simulink model "Hybrid_PV_Wind_Subsystem"  (R2018a)
settings: Solver=ode5  StartTime=0.0  StopTime=10  RelTol=1e-3
PreLoadFcn:
  | Ts_Power=1e-6;
  | Ts_Control=100e-6;
undefined symbols (not defined in the file): D1, Delta, DiscIntNeverNeededParam, sigbuilder_block
libraries: powerlib x32, powerlib_meascontrol x11, re_lib x2, simulink x2
(part 1 of 2)
Description:
  | Copyright 2008-2018 The MathWorks, Inc.
settings Model: SimulationMode=accelerator  Creator=MathWorks  LastModifiedBy=ASUS
settings DataIOCC: LimitDataPoints=on  SaveFormat=Array  SignalLoggingSaveFormat=ModelDataLogs  SignalLogging=off  DSMLogging=off
settings OptimizationCC: ExpressionDepthLimit=2147483647  EfficientMapNaN2IntZero=off  LifeSpan=inf
settings DebuggingCC: UnderspecifiedInitializationDetection=Classic  MergeDetectMultiDrivingBlocksExec=none  SolverPrmCheckMsg=warning  FcnCallInpInsideContextMsg=warning  StateNameClashWarn=warning  LibraryContextMissingDiagnostic=warning  SFUnexpectedBacktrackingDiag=warning  SFNoUnconditionalDefaultTransitionDiag=warning  SFExecutionAtInitializationDiag=none
settings HardwareCC: ProdBitPerPointer=32  ProdBitPerSizeT=32  ProdBitPerPtrDiffT=32  ProdLargestAtomicFloat=None  ProdIntDivRoundTo=Undefined  ProdEndianess=Unspecified  ProdWordSize=32  ProdHWDeviceType=32-bit Generic  TargetBitPerPointer=64  TargetBitPerSizeT=64  TargetBitPerPtrDiffT=64  TargetLongLongMode=on  TargetIntDivRoundTo=Zero  TargetEndianess=LittleEndian  TargetWordSize=64  TargetHWDeviceType=MATLAB Host  ProdEqTarget=off
settings ModelReferenceCC: PropagateSignalLabelsOutOfModel=off
settings RTWCC: RTWUseLocalCustomCode=on
settings CodeAppCC: MaxIdLength=128
settings GRTTargetCC: TargetLangStandard=C89/C90 (ANSI)  CombineOutputUpdateFcns=off  GRTInterface=on
settings ConfigComp: CovMetricSettings=dw  CovHtmlReporting=on  CovSaveCumulativeToWorkspaceVar=on  CovSaveSingleToWorkspaceVar=on  CovExternalEMLEnable=off  CovSFcnEnable=off
settings SimscapeCC: SimscapeNormalizeSystem=off

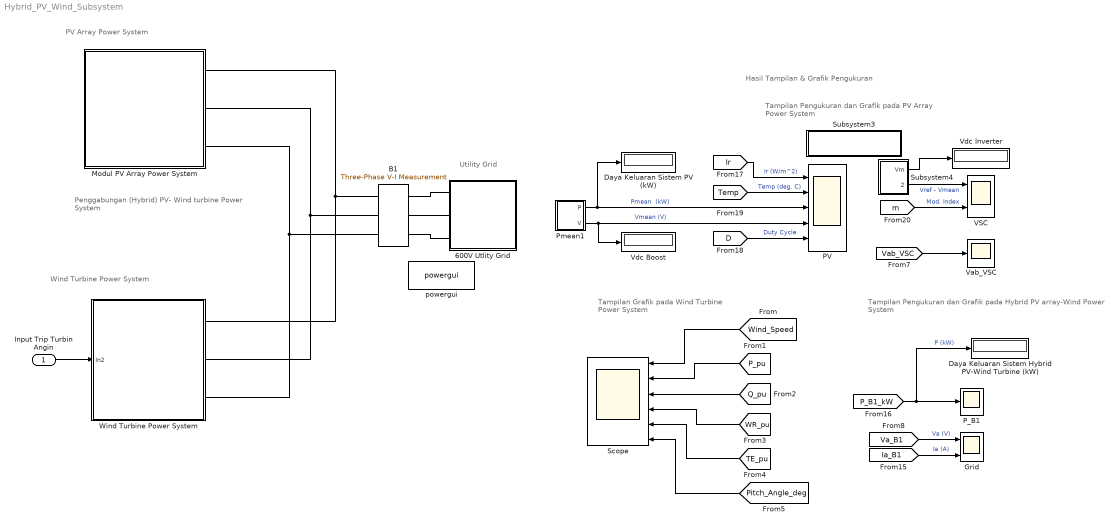
== system Hybrid_PV_Wind_Subsystem ==
  note: Hasil Tampilan & Grafik Pengukuran
  note: Penggabungan
      | (Hybrid) PV- Wind turbine
      | Power System
  note: Tampilan Grafik pada
      | Wind Turbine Power System
  note: PV Array Power System
  note: Wind Turbine Power System
  note: Tampilan Pengukuran dan
      | Grafik pada PV Array Power System
  note: Tampilan Pengukuran dan
      | Grafik pada Hybrid PV array-Wind Power System
  note: Utility Grid
  Input Trip Turbin Angin : Inport
  " Modul PV Array Power System" : Subsystem
  " Wind Turbine Power System" : Subsystem
  600V Utlity Grid : Subsystem
      mask Display: image(imread('grid.jpg'))
  B1 : powerlib/Measurements/Three-Phase V-I Measurement  VoltageMeasurement=phase-to-ground  SetLabelV=on  LabelV=Vabc_B1  Vpu=off  VpuLL=off  CurrentMeasurement=yes  SetLabelI=on  LabelI=Iabc_B1  Ipu=off  Pbase=100e6  Vbase=500e3  OutputType=Magnitude  PhasorSimulation=on  PSBequivalent=0
      settings: SourceProductName=Simscape Electrical
  Daya Keluaran Sistem Hybrid PV-Wind Turbine (kW) : Display
      settings: Format=bank  Decimation=2000
  "Daya Keluaran Sistem PV (kW) " : Display
      settings: Format=bank  Decimation=2000
  Grid : Scope  NumInputPorts=2
  PV : Scope  NumInputPorts=5
  P_B1 : Scope
  Pmean1 : Subsystem
  Scope : Scope  NumInputPorts=6
  Subsystem3 : Subsystem
      mask Display: disp('Open this block\nto display additional \nscopes & measurements')
  Subsystem4 : Subsystem
  VSC : Scope  NumInputPorts=2
  Vab_VSC : Scope
  Vdc Boost : Display
      settings: Format=bank  Decimation=2000
  Vdc Inverter : Display
      settings: Format=bank  Decimation=2000
  powergui : powerlib/powergui  Priority=1  SimulationMode=Discrete  SampleTime=Ts_Power  frequency=60  Iterations=50  frequencyindice=0  Pbase=100e6  ErrMax=1e-4  UnitsV=kV  UnitsW=MW  buscounter=0  FunctionMessages=off  echomessages=off  EnableUseOfTLC=off  CurrentSourceSwitches=off  DisableSnubberDevices=off  DisableRonSwitches=off  DisableVfSwitches=off  DisplayEquations=off  SolverType=Tustin/Backward Euler (TBE)  Interpol=off  ExternalGateDelay=off  methode=off  Ts=0  x0status=blocks  SPID=off  SwTol=0  HookPort=off  RestoreLinks=warning  ResistiveCurrentMeasurement=off  Frange=[0:2:500]  Ylog=off  Xlog=on  ShowGrid=off  save=off  variable=ZData  structure=0  ZoomFFT=on  StartTime=0.0  cycles=1  DisplayStyle=1  fundamental=60  FreqAxis=off  MaxFrequency=1000  frequencyindicesteady=1  RmsSteady=1  display=off
  wires:
  Subsystem4/2(VrVm) -> VSC/1  "Vref - Vmean"
  Pmean1/1(P) -> "Daya Keluaran Sistem PV (kW) "/1, PV/3  "Pmean  (kW)"
  [Ir] -> PV/1  "Ir (W/m^2)"
  [Ia_B1] -> Grid/2  "Ia (A)"
  [Temp] -> PV/2  "Temp (deg. C)"
  [Va_B1] -> Grid/1  "Va (V)"
  Pmean1/2(V) -> Vdc Boost/1, PV/4  "Vmean (V)"
  [D] -> PV/5  "Duty Cycle"
  [P_B1_kW] -> P_B1/1, Daya Keluaran Sistem Hybrid PV-Wind Turbine (kW)/1  "P (kW)"
  [Vab_VSC] -> Vab_VSC/1
  [m] -> VSC/2  "Mod. Index"
  Subsystem4/1(Vm) -> Vdc Inverter/1
  Input Trip Turbin Angin/1 -> " Wind Turbine Power System"/1(In2)
  [Wind_Speed] -> Scope/1
  [P_pu] -> Scope/2
  [Q_pu] -> Scope/3
  [WR_pu] -> Scope/4
  [TE_pu] -> Scope/5
  [Pitch_Angle_deg] -> Scope/6
  connections:
  B1/RConn3 -- 600V Utlity Grid/LConn3
  B1/RConn2 -- 600V Utlity Grid/LConn2
  B1/RConn1 -- 600V Utlity Grid/LConn1
  " Modul PV Array Power System"/RConn1 -- " Wind Turbine Power System"/RConn1 -- B1/LConn1
  " Modul PV Array Power System"/RConn2 -- " Wind Turbine Power System"/RConn2 -- B1/LConn2
  " Modul PV Array Power System"/RConn3 -- " Wind Turbine Power System"/RConn3 -- B1/LConn3

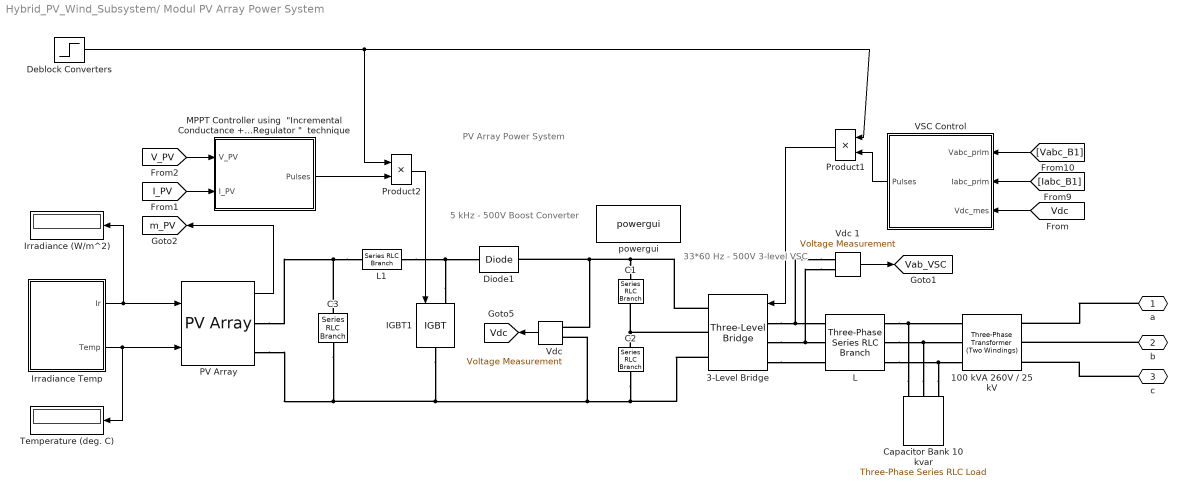
== system Hybrid_PV_Wind_Subsystem/ Modul PV Array Power System ==
  note: 5 kHz - 500V
      | Boost Converter
  note: 33*60 Hz - 500V
      | 3-level VSC
  note: PV Array Power System
  100 kVA 260V / 25 kV : powerlib/Elements/Three-Phase Transformer (Two Windings)  Winding1Connection=Yg  Winding2Connection=Delta (D1)  CoreType=Three single-phase transformers  SetSaturation=off  Hysteresis=off  DataFile='hysteresis'  SetInitialFlux=off  Measurements=None  UNITS=pu  NominalPower=[100e3 , 60 ]  Winding1=[ 25e3 , 0.001 , 0.03 ]  Winding2=[ 260 , 0.001 , 0.03 ]  Rm=500  Lm=500  L0=0.5  Saturation=[ 0,0 ; 0.0024,1.2 ; 1.0,1.52 ]  InitialFluxes=[ 0.8 , -0.8 , 0.7 ]  MoreParameters=off  BreakLoop=off  DataType=off  TransfoNumber=0
      settings: SourceProductName=Simscape Electrical
  3-Level Bridge : powerlib/Power Electronics/Three-Level Bridge  Arms=3  SnubberResistance=1e6  SbubberCapacitance=inf  Device=IGBT / Diodes  Ron=0.2e-3  ForwardVoltages="[  0  0 ]"  Measurements=None
      settings: SourceProductName=Simscape Electrical  SourceProductBaseCode=PS
  C1 : powerlib/Elements/Series RLC Branch  LConnTagsString=__new0  RConnTagsString=__new0  BranchType=C  Resistance=1.0  Inductance=1.0  SetiL0=off  InitialCurrent=0  Capacitance=12000e-06  Setx0=off  InitialVoltage=0  Measurements=None
      settings: SourceProductName=Simscape Electrical
  C2 : powerlib/Elements/Series RLC Branch  LConnTagsString=__new0  RConnTagsString=__new0  BranchType=C  Resistance=1.0  Inductance=1.0  SetiL0=off  InitialCurrent=0  Capacitance=12000e-06  Setx0=off  InitialVoltage=0  Measurements=None
      settings: SourceProductName=Simscape Electrical
  C3 : powerlib/Elements/Series RLC Branch  LConnTagsString=__new0  RConnTagsString=__new0  BranchType=C  Resistance=1.0  Inductance=1.0  SetiL0=off  InitialCurrent=0  Capacitance=100e-6  Setx0=off  InitialVoltage=0  Measurements=Branch voltage
      settings: SourceProductName=Simscape Electrical
  Capacitor Bank 10 kvar : powerlib/Elements/Three-Phase Series RLC Load  LConnTagsString=A|B|C  Configuration=Y (grounded)  NominalVoltage=240  Vabc=[1e3 1e3 1e3]  Vabcp=[1e3 1e3 1e3]  NominalFrequency=60  UnbalancedPower=off  ActivePower=10e3/100  InductivePower=0  CapacitivePower=10e3  Pabc=[10e3 9e3 11e3]  QLabc=[100 90 110]  QCabc=[100 90 110]  Pabcp=[10e3 9e3 11e3]  QLabcp=[100 90 110]  QCabcp=[100 90 110]  Measurements=None  LoadType=constant Z
      settings: SourceProductName=Simscape Electrical
  Deblock Converters : Step  Time=0.05  SampleTime=0
  Diode1 : powerlib/Power Electronics/Diode  Ron=1e-4  Lon=0  Vf=0  IC=0  UseSnubber=off  Rs=inf  Cs=inf  Measurements=off
      settings: SourceProductName=Simscape Electrical
  IGBT1 : powerlib/Power Electronics/IGBT  Ron=0.001  Lon=0  Vf=0  Tf=0  Tt=0  IC=0  Rs=1e5  Cs=inf  Measurements=off
      settings: SourceProductName=Simscape Electrical
  Irradiance (W/m^2) : Display
      settings: Format=bank  Decimation=1000
  Irradiance Temp : Subsystem  Tag=STV Subsys  LoadFcn=sigbuilder_block('load');  StartFcn=sigbuilder_block('start');  StopFcn=sigbuilder_block('stop');  ClipboardFcn=sigbuilder_block('clipboard');  mask(Sigbuilder block){tuvar=[0:10]}
      mask help: Sigbuilder GUI
      mask init:
      | if ~strcmp(get_param(bdroot(gcbh),'SimulationStatus'),'stopped') tuvar = sigbuilder_block('maskInit'); end
      settings: CopyFcn=sigbuilder_block('copy');  DeleteFcn=sigbuilder_block('delete');  ModelCloseFcn=sigbuilder_block('modelClose');  PreSaveFcn=sigbuilder_block('preSave');  PauseFcn=sigbuilder_block('pause')  ContinueFcn=sigbuilder_block('continue')  NameChangeFcn=sigbuilder_block('namechange');  OpenFcn=sigbuilder_block('open',[216.75 77.25 531 395.25 ]);  CloseFcn=sigbuilder_block('close');
      mask Display: plot(0, 0, 100, 100,[2, 2, 32, 32, 2], [68, 8, 8, 68, 68],[32, 2], [38, 38], [32, 19, 2],[53, 60, 44], [32, 17, 17, 2],[16, 16, 31, 31]);txt = getActiveGroup(gcbh);text(2, 100, txt,'verticalAlignment', 'top');
  L : powerlib/Elements/Three-Phase Series RLC Branch  LConnTagsString=A|B|C  RConnTagsString=A|B|C  BranchType=RL  Resistance=500e-6*377/50/2  Inductance=500e-6/2  Capacitance=inf  Measurements=None
      settings: SourceProductName=Simscape Electrical
  L1 : powerlib/Elements/Series RLC Branch  LConnTagsString=__new0  RConnTagsString=__new0  BranchType=RL  Resistance=0.005  Inductance=5e-3  SetiL0=off  InitialCurrent=0  Capacitance=1e-6  Setx0=off  InitialVoltage=0  Measurements=None
      settings: SourceProductName=Simscape Electrical
  "MPPT Controller using  \"Incremental Conductance + Integral Regulator \"  technique " : Subsystem  mask(Boost Control - MPPT){fc=5000, T_MPPT=200e-6, Dinit=0.5}
      mask prompts: fc "PWM switching frequency (Hz)"; T_MPPT "Time window used by MPPT control (s)"; Dinit "Initial value of duty cycle"
  PV Array : re_lib/Solar/PV Array  Npar=9  Nser=5  PlotType=array @ 1000 W/m2 & specified temperatures  S_vec="[ 1000  250 ]"  Temp_C_vec="[0 25 50  ]"  ModuleName=SunPower SPR-305E-WHT-D  PlotWhenSelected=off  Pm=305.226  Ncell=96  Voc=64.2  Isc=5.96  Vm=54.7  Im=5.58  beta_Voc_pc=-0.27269  alpha_Isc_pc=0.061745  beta_Voc=-0.17507  alpha_Isc=0.00368  IL=6.0092  I0=6.3014e-12  nI=0.94504  Rsh=269.5934  Rs=0.37152  BAL=on  Tc=Tc  Tfilter=5e-5
      settings: SourceProductName=Simscape Electrical
  Product1 : Product  RndMeth=Zero
  Product2 : Product  RndMeth=Zero
  Temperature (deg. C) : Display
      settings: Format=bank  Decimation=1000
  VSC Control : Subsystem  mask(VSC Main Controller){nom=[ 100e3  60 ], Vnom=[ 25e3 260 ], Vnom_dc=500, RLxfo=[0.002  0.06 ], RLchoke=[2e-3  250e-6  ], K_VDCreg=[7  800], K_Ireg=[0.3 20], Ts=Ts_Control}
      mask prompts: nom "Nominal power and frequency [ Pnom(VA)  Fnom(Hz) ]:"; Vnom "Nominal primary and secondary voltages (Vrms LL) [ Vnom_prim   Vnom_sec ]:"; Vnom_dc "Nominal DC bus voltage (V):"; RLxfo "Total transformer leakage impedance (pu/Pnom) [ Rxfo  Lxf ]"; RLchoke "Choke impedance [ R(ohm) L(H) ]"; K_VDCreg "VDC regultator gains [ Kp  Ki ]:"; K_Ireg "Current regulator gains [ Kp  Ki ]:"; Ts "Sample time"
      mask init:
      | Pnom=nom(1);
      | Fnom=nom(2);
      | Vnom_prim=Vnom(1);
      | Vnom_sec=Vnom(2);
      | Zbase=Vnom_sec^2/Pnom;
      | Rtot_pu=RLxfo(1) + RLchoke(1)/Zbase;
      | Ltot_pu=RLxfo(2) + RLchoke(2)/(Zbase/(2*pi*Fnom));
      | Kp_VDCreg=K_VDCreg(1);
      | Ki_VDCreg=K_VDCreg(2);
      | Kp_Ireg=K_Ireg(1);
      | Ki_Ireg=K_Ireg(2);
      | Vdc_ref=Vnom_dc;
      | % Used to determine initial value of Boost Control (MPPT)
      | assignin('base','Vdc_ref_Inv',Vdc_ref);
  "Vdc " : powerlib/Measurements/Voltage Measurement  Tag=PoWeRsYsTeMmEaSuReMeNt  PhasorSimulation=off  OutputType=Magnitude  PSBequivalent=0
      settings: SourceProductName=Simscape Electrical
  Vdc 1 : powerlib/Measurements/Voltage Measurement  Tag=PoWeRsYsTeMmEaSuReMeNt  PhasorSimulation=off  OutputType=Magnitude  PSBequivalent=0
      settings: SourceProductName=Simscape Electrical
  powergui : powerlib/powergui  Priority=1  SimulationMode=Discrete  SampleTime=Ts_Power  frequency=60  Iterations=50  frequencyindice=0  Pbase=100e6  ErrMax=1e-4  UnitsV=kV  UnitsW=MW  buscounter=0  FunctionMessages=off  echomessages=off  EnableUseOfTLC=off  CurrentSourceSwitches=off  DisableSnubberDevices=off  DisableRonSwitches=off  DisableVfSwitches=off  DisplayEquations=off  SolverType=Tustin/Backward Euler (TBE)  Interpol=off  ExternalGateDelay=off  methode=off  Ts=0  x0status=blocks  SPID=off  SwTol=0  HookPort=off  RestoreLinks=warning  ResistiveCurrentMeasurement=off  Frange=[0:2:500]  Ylog=off  Xlog=on  ShowGrid=off  save=off  variable=ZData  structure=0  ZoomFFT=on  StartTime=0.0  cycles=1  DisplayStyle=1  fundamental=60  FreqAxis=off  MaxFrequency=1000  frequencyindicesteady=1  RmsSteady=1  display=off
      settings: SourceProductName=Simscape Electrical
  a : PMIOPort  Side=Right
  b : PMIOPort  Port=2  Side=Right
  c : PMIOPort  Port=3  Side=Right
  tag scope: Vab_VSC=global, Vdc=global, m_PV=global
  wires:
  Vdc 1/1 -> [Vab_VSC]
  [I_PV] -> "MPPT Controller using  \"Incremental Conductance + Integral Regulator \"  technique "/2(I_PV)
  Product1/1 -> 3-Level Bridge/1
  Irradiance Temp/2(Temp) -> PV Array/2, Temperature (deg. C)/1
  Deblock Converters/1 -> Product2/1, Product1/1
  [Vabc_B1] -> VSC Control/1(Vabc_prim)
  "Vdc "/1 -> [Vdc]
  [Vdc] -> VSC Control/3(Vdc_mes)
  [V_PV] -> "MPPT Controller using  \"Incremental Conductance + Integral Regulator \"  technique "/1(V_PV)
  "MPPT Controller using  \"Incremental Conductance + Integral Regulator \"  technique "/1(Pulses) -> Product2/2
  Product2/1 -> IGBT1/1
  Irradiance Temp/1(Ir) -> PV Array/1, Irradiance (W/m^2)/1
  PV Array/1 -> [m_PV]
  VSC Control/1(Pulses) -> Product1/2
  [Iabc_B1] -> VSC Control/2(Iabc_prim)
  connections:
  3-Level Bridge/RConn2 -- C2/LConn1 -- C1/RConn1
  L1/LConn1 -- C3/LConn1 -- PV Array/RConn1
  Capacitor Bank 10 kvar/LConn2 -- L/RConn2 -- 100 kVA 260V / 25 kV/RConn2
  C2/RConn1 -- PV Array/RConn2 -- C3/RConn1 -- IGBT1/RConn1 -- "Vdc "/LConn2 -- 3-Level Bridge/RConn3
  Vdc 1/LConn1 -- 3-Level Bridge/LConn1 -- L/LConn1
  IGBT1/LConn1 -- L1/RConn1 -- Diode1/LConn1
  Vdc 1/LConn2 -- 3-Level Bridge/LConn2 -- L/LConn2
  Capacitor Bank 10 kvar/LConn3 -- L/RConn3 -- 100 kVA 260V / 25 kV/RConn3
  C1/LConn1 -- 3-Level Bridge/RConn1 -- Diode1/RConn1 -- "Vdc "/LConn1
  Capacitor Bank 10 kvar/LConn1 -- L/RConn1 -- 100 kVA 260V / 25 kV/RConn1
  3-Level Bridge/LConn3 -- L/LConn3
  a/RConn1 -- 100 kVA 260V / 25 kV/LConn1
  b/RConn1 -- 100 kVA 260V / 25 kV/LConn2
  c/RConn1 -- 100 kVA 260V / 25 kV/LConn3

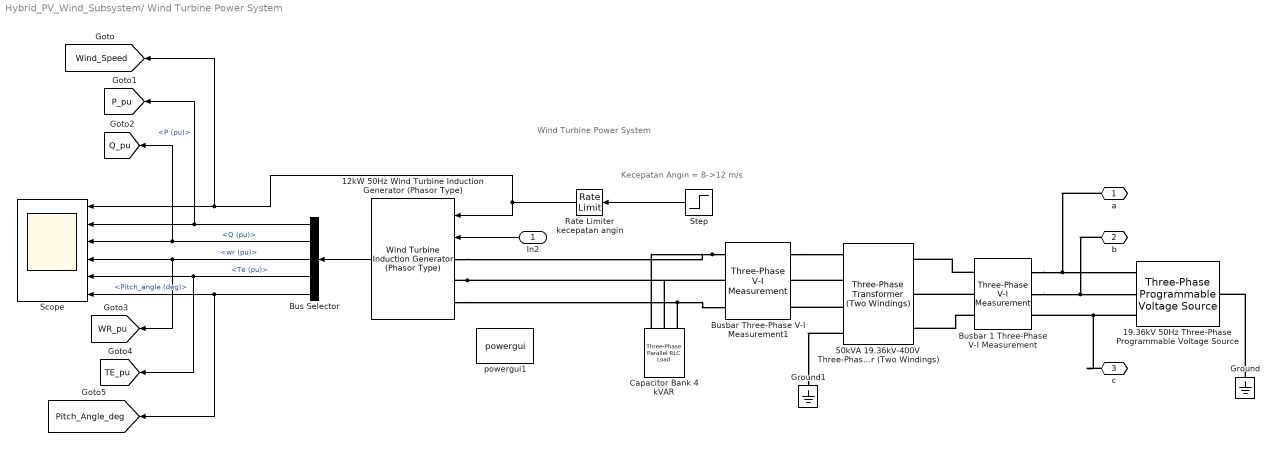
== system Hybrid_PV_Wind_Subsystem/ Wind Turbine Power System ==
  note: Wind Turbine Power System
  note: Kecepatan Angin = 8->12 m/s
  In2 : Inport
  12kW 50Hz Wind Turbine Induction Generator (Phasor Type) : re_lib/Wind Generation/Wind Turbine Induction Generator (Phasor Type)  ExternalTm=off  nom=[12e3, 400, 50]  sta=[ 0.004843, 0.1248]  rot=[ 0.004377, 0.1791]  Lm=6.77  mec=[5.04, 0.01, 3]  init="[ -0.01,0,   0,0,0,   0,0,0 ]"  pitch_angle=0  Pmec=12e3  wind_base=12  speed_nom=1  P_wind_base=1  K_pitch_gain=[5 25]  pitch_max=45  pitch_rate=2
      settings: SourceProductName=Simscape Electrical  SourceProductBaseCode=PS
  19.36kV 50Hz Three-Phase Programmable Voltage Source : powerlib/Electrical Sources/Three-Phase Programmable Voltage Source  PositiveSequence="[19.36e3  0 50]"  VariationEntity=None  VariationType=Table of time-amplitude pairs  VariationTypeAlt=Step  VariationStep=0.5  VariationRate=10  VariationMagnitude=0.3  VariationFrequency=2  VariationTiming=[1 2]  VariationPhaseA=off  Amplitudes=[1 0.8 1.2 1.0]  TimeValues=[0 0.1 0.15 0.2]  HarmonicGeneration=off  HarmonicA=[3 0.2 -25 0]  HarmonicB=[2 0.15 35 2]  Timing="[0.05  3]"  BusType=swing  Pref=0  Qref=0  Qmin=-inf  Qmax=inf
      settings: SourceProductName=Simscape Electrical
  50kVA 19.36kV-400V Three-Phase Transformer (Two Windings) : powerlib/Elements/Three-Phase Transformer (Two Windings)  Winding1Connection=Yg  Winding2Connection=Yn  CoreType=Three single-phase transformers  SetSaturation=off  Hysteresis=off  DataFile='hysteresis'  SetInitialFlux=off  Measurements=None  UNITS=pu  NominalPower=[ 50e3 , 50 ]  Winding1=[ 19.36e3 , 0.002 , 0.08 ]  Winding2=[ 400 , 0.002 , 0.08 ]  Rm=500  Lm=inf  L0=0.5  Saturation=[ 0,0 ; 0.0024,1.2 ; 1.0,1.52 ]  InitialFluxes=[ 0.8 , -0.8 , 0.7 ]  MoreParameters=off  BreakLoop=off  DataType=off  TransfoNumber=1
      settings: SourceProductName=Simscape Electrical
  Bus Selector : BusSelector  OutputSignals=P (pu),Q (pu),wr (pu),Te (pu),Pitch_angle (deg)
  Busbar 1 Three-Phase V-I Measurement : powerlib/Measurements/Three-Phase V-I Measurement  VoltageMeasurement=phase-to-ground  SetLabelV=on  LabelV=Vabc  Vpu=off  VpuLL=off  CurrentMeasurement=yes  SetLabelI=on  LabelI=Iabc  Ipu=off  Pbase=100e6  Vbase=500e3  OutputType=Complex  PhasorSimulation=on  PSBequivalent=0
      settings: SourceProductName=Simscape Electrical
  Busbar Three-Phase V-I Measurement1 : powerlib/Measurements/Three-Phase V-I Measurement  VoltageMeasurement=phase-to-ground  SetLabelV=on  LabelV=WTVabc  Vpu=off  VpuLL=off  CurrentMeasurement=yes  SetLabelI=on  LabelI=WTIabc  Ipu=off  Pbase=100e6  Vbase=500e3  OutputType=Complex  PhasorSimulation=on  PSBequivalent=0
      settings: SourceProductName=Simscape Electrical
  Capacitor Bank 4 kVAR : powerlib/Elements/Three-Phase Parallel RLC Load  LConnTagsString=A|B|C  Configuration=Y (grounded)  NominalVoltage=400  Vabc=[1e3 1e3 1e3]  Vabcp=[1e3 1e3 1e3]  NominalFrequency=50  UnbalancedPower=off  ActivePower=0  InductivePower=0  CapacitivePower=4e3  Pabc=[10e3 9e3 11e3]  QLabc=[100 90 110]  QCabc=[100 90 110]  Pabcp=[10e3 9e3 11e3]  QLabcp=[100 90 110]  QCabcp=[100 90 110]  Measurements=None  LoadType=constant Z
      settings: SourceProductName=Simscape Electrical
  Ground : powerlib/Elements/Ground  LConnTagsString=a
      settings: SourceProductName=Simscape Electrical
  Ground1 : powerlib/Elements/Ground  LConnTagsString=a
      settings: SourceProductName=Simscape Electrical
  "Rate Limiter kecepatan angin " : RateLimiter
  Scope : Scope  NumInputPorts=6
  Step : Step  Time=5  Before=8  After=12  SampleTime=0
  powergui1 : powerlib/powergui  Priority=1  SimulationMode=Phasor  SampleTime=50e-6  frequency=50  Iterations=50  frequencyindice=50  Pbase=100e6  ErrMax=1e-4  UnitsV=kV  UnitsW=MW  buscounter=0  FunctionMessages=off  echomessages=off  EnableUseOfTLC=off  CurrentSourceSwitches=off  DisableSnubberDevices=off  DisableRonSwitches=off  DisableVfSwitches=off  DisplayEquations=off  SolverType=Tustin/Backward Euler (TBE)  Interpol=off  ExternalGateDelay=off  methode=off  Ts=100  x0status=blocks  SPID=off  SwTol=0  HookPort=off  RestoreLinks=warning  ResistiveCurrentMeasurement=off  Frange=[0:2:500]  Ylog=off  Xlog=on  ShowGrid=off  save=off  variable=ZData  structure=0  ZoomFFT=off  StartTime=0.0  cycles=1  DisplayStyle=1  fundamental=60  FreqAxis=off  MaxFrequency=1000  frequencyindicesteady=1  RmsSteady=1  display=off
      settings: SourceProductName=Simscape Electrical
  a : PMIOPort  Side=Right
  b : PMIOPort  Port=2  Side=Right
  c : PMIOPort  Port=3  Side=Right
  tag scope: P_pu=global, Pitch_Angle_deg=global, Q_pu=global, TE_pu=global, WR_pu=global, Wind_Speed=global
  wires:
  12kW 50Hz Wind Turbine Induction Generator (Phasor Type)/1 -> Bus Selector/1
  Step/1 -> "Rate Limiter kecepatan angin "/1
  "Rate Limiter kecepatan angin "/1 -> 12kW 50Hz Wind Turbine Induction Generator (Phasor Type)/1, [Wind_Speed], Scope/1
  Bus Selector/1 -> [P_pu], Scope/2  "<P (pu)>"
  Bus Selector/3 -> [WR_pu], Scope/4  "<wr (pu)>"
  Bus Selector/2 -> [Q_pu], Scope/3  "<Q (pu)>"
  In2/1 -> 12kW 50Hz Wind Turbine Induction Generator (Phasor Type)/2
  Bus Selector/4 -> [TE_pu], Scope/5  "<Te (pu)>"
  Bus Selector/5 -> [Pitch_Angle_deg], Scope/6  "<Pitch_angle (deg)>"
  connections:
  12kW 50Hz Wind Turbine Induction Generator (Phasor Type)/LConn2 -- Busbar Three-Phase V-I Measurement1/RConn2 -- Capacitor Bank 4 kVAR/LConn2
  Busbar Three-Phase V-I Measurement1/RConn1 -- 12kW 50Hz Wind Turbine Induction Generator (Phasor Type)/LConn1 -- Capacitor Bank 4 kVAR/LConn1
  Capacitor Bank 4 kVAR/LConn3 -- 12kW 50Hz Wind Turbine Induction Generator (Phasor Type)/LConn3 -- Busbar Three-Phase V-I Measurement1/RConn3
  Busbar Three-Phase V-I Measurement1/LConn1 -- 50kVA 19.36kV-400V Three-Phase Transformer (Two Windings)/RConn1
  Busbar 1 Three-Phase V-I Measurement/RConn2 -- 50kVA 19.36kV-400V Three-Phase Transformer (Two Windings)/LConn2
  19.36kV 50Hz Three-Phase Programmable Voltage Source/RConn3 -- c/RConn1 -- Busbar 1 Three-Phase V-I Measurement/LConn3
  Busbar 1 Three-Phase V-I Measurement/RConn3 -- 50kVA 19.36kV-400V Three-Phase Transformer (Two Windings)/LConn3
  Busbar 1 Three-Phase V-I Measurement/LConn1 -- a/RConn1 -- 19.36kV 50Hz Three-Phase Programmable Voltage Source/RConn1
  Busbar 1 Three-Phase V-I Measurement/LConn2 -- 19.36kV 50Hz Three-Phase Programmable Voltage Source/RConn2 -- b/RConn1
  Ground/LConn1 -- 19.36kV 50Hz Three-Phase Programmable Voltage Source/LConn1
  50kVA 19.36kV-400V Three-Phase Transformer (Two Windings)/RConn2 -- Busbar Three-Phase V-I Measurement1/LConn2
  50kVA 19.36kV-400V Three-Phase Transformer (Two Windings)/RConn4 -- Ground1/LConn1
  50kVA 19.36kV-400V Three-Phase Transformer (Two Windings)/RConn3 -- Busbar Three-Phase V-I Measurement1/LConn3
  Busbar 1 Three-Phase V-I Measurement/RConn1 -- 50kVA 19.36kV-400V Three-Phase Transformer (Two Windings)/LConn1

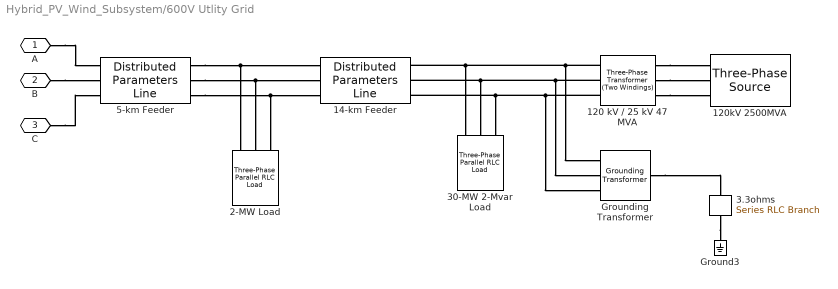
== system Hybrid_PV_Wind_Subsystem/600V Utlity Grid ==
  120 kV / 25 kV 47 MVA : powerlib/Elements/Three-Phase Transformer (Two Windings)  Winding1Connection=Yg  Winding2Connection=Delta (D1)  CoreType=Three single-phase transformers  SetSaturation=off  Hysteresis=off  DataFile='basic_model'  SetInitialFlux=off  Measurements=None  UNITS=pu  NominalPower=[47e6 60 ]  Winding1="[ 120e3  0.08/30   0.08 ]"  Winding2="[ 25e3  0.08/30  0.08]"  Rm=500  Lm=500  L0=0.5  Saturation="[ 0,0  ;  0.005,1.2  ;  1.0,1.4 ]"  InitialFluxes=[ 0.8 , -0.8 , 0.7 ]  MoreParameters=off  BreakLoop=off  DataType=off  TransfoNumber=0
      settings: SourceProductName=Simscape Electrical
  120kV 2500MVA : powerlib/Electrical Sources/Three-Phase Source  InternalConnection=Yg  VoltagePhases=off  Voltage=120e3  PhaseAngle=0  Voltage_phases=[25e3 25e3 25e3]/sqrt(3)  PhaseAngles_phases=[0 -120 +120]  Frequency=60  NonIdealSource=on  SpecifyImpedance=on  Resistance=0.8929  Inductance=16.58e-3  ShortCircuitLevel=2500e6  BaseVoltage=120e3  XRratio=7  BusType=swing  Pref=0  Qref=0  Prefabc=[10e3, 10e3, 10e3]  Qrefabc=[0, 0, 0]  Qmin=-inf  Qmax=inf
      settings: SourceProductName=Simscape Electrical
  14-km Feeder : powerlib/Elements/Distributed Parameters Line  Phases=3  Frequency=60  Resistance=[0.1153 0.413]  Inductance=[1.05e-3 3.32e-3]  Capacitance=[11.33e-009 5.01e-009]  Length=14  x1=[-5.8e-05 -3.3791322040864e-10 0 0;-5.7e-05 -3.37999167380001e-10 0 0;-5.6e-05 -3.38085103385797e-10 0 0;-5.5e-05 -3.38171028409331e-10 0 0;-5.4e-05 -3.38256942433901e-10 0 0;-5.3e-05 -3.38342845442808e-10 0 0;-5.2e-05 -3.38428737419346e-10 0 0;-5.1e-05 -3.38514618346809e-10 0 0;-5e-05 -3.3860048820849e-10 0 0;-4.9e-05 -3.38686346987679e-10 6763.35570826325 -18298.0571778383;-4.8e-05 -3.38772194667662e-10 6769.41188071272 -18295.9827223402;-4.7e-05 -3.38858031231726e-10 6775.46742044088 -18293.9062482242;-4.6e-05 -3.38943856663154e-10 6781.52232676982 -18291.8277556818;-4.5e-05 -3.39029670945228e-10 6787.57659902169 -18289.7472449049;-4.4e-05 -3.39115474061227e-10 6793.63023651868 -18287.6647160855;-4.3e-05 -3.39201265994428e-10 6799.68323858306 -18285.580169416;-4.2e-05 -3.39287046728108e-10 6805.73560453714 -18283.4936050888;-4.1e-05 -3.39372816245538e-10 6811.7873337033 -18281.4050232968;-4e-05 -3.3945857452999e-10 6817.83842540397 -18279.3144242329;-3.9e-05 -3.39544321564734e-10 6823.88887896164 -18277.2218080903;-3.8e-05 -3.39630057333036e-10 6829.93869369886 -18275.1271750626;-3.7e-05 -3.39715781818161e-10 6835.98786893825 -18273.0305253433;-3.6e-05 -3.39801495003372e-10 6842.03640400246 -18270.9318591263;-3.5e-05 -3.39887196871931e-10 6848.08429821421 -18268.8311766059;-3.4e-05 -3.39972887407096e-10 6854.1315508963 -18266.7284779764;-3.3e-05 -3.40058566592124e-10 6860.17816137155 -18264.6237634323;-3.2e-05 -3.4014423441027e-10 6866.22412896288 -18262.5170331685;-3.1e-05 -3.40229890844786e-10 6872.26945299323 -18260.40828738;-3e-05 -3.40315535878924e-10 6878.31413278563 -18258.2975262622;-2.9e-05 -3.40401169495931e-10 6884.35816766314 -18256.1847500105;-2.8e-05 -3.40486791679056e-10 6890.40155694891 -18254.0699588206;-2.7e-05 -3.40572402411541e-10 6896.44429996612 -18251.9531528886;-2.6e-05 -3.40658001676631e-10 6902.48639603803 -18249.8343324107;-2.5e-05 -3.40743589457565e-10 6908.52784448795 -18247.7134975832;-2.4e-05 -3.40829165737583e-10 6914.56864463925 -18245.5906486029;-2.3e-05 -3.40914730499921e-10 6920.60879581535 -18243.4657856665;-2.2e-05 -3.41000283727813e-10 6926.64829733975 -18241.3389089713;-2.1e-05 -3.41085825404493e-10 6932.68714853599 -18239.2100187145;-2e-05 -3.4117135551319e-10 6938.72534872768 -18237.0791150938;-1.9e-05 -3.41256874037133e-10 6944.76289723849 -18234.9461983069;-1.8e-05 -3.4134238095955e-10 6950.79979339215 -18232.8112685519;-1.7e-05 -3.41427876263664e-10 6956.83603651243 -18230.674326027;-1.6e-05 -3.41513359932698e-10 6962.87162592319 -18228.5353709308;-1.5e-05 -3.41598831949874e-10 6968.90656094833 -18226.3944034619;-1.4e-05 -3.41684292298408e-10 6974.94084091182 -18224.2514238192;-1.3e-05 -3.41769740961519e-10 6980.97446513768 -18222.1064322021;-1.2e-05 -3.41855177922421e-10 6987.00743295 -18219.9594288098;-1.1e-05 -3.41940603164327e-10 6993.03974367293 -18217.810413842;-1e-05 -3.42026016670447e-10 6999.07139663066 -18215.6593874985;-9e-06 -3.4211141842399e-10 7005.10239114747 -18213.5063499795;-8e-06 -3.42196808408162e-10 7011.13272654769 -18211.3513014853;-7e-06 -3.4228218660617e-10 7017.1624021557 -18209.1942422164;-6e-06 -3.42367553001215e-10 7023.19141729595 -18207.0351723736;-5e-06 -3.42452907576499e-10 7029.21977129294 -18204.8740921578;-4e-06 -3.42538250315221e-10 7035.24746347125 -18202.7110017705;-3e-06 -3.42623581200577e-10 7041.27449315551 -18200.5459014129;-2e-06 -3.42708900215763e-10 7047.3008596704 -18198.3787912868;-1e-06 -3.42794207343972e-10 7053.32656234069 -18196.2096715941]  x2=[-5.8e-05 -1.48060604917725e-09 0 0;-5.7e-05 -1.4809460705246e-09 0 0;-5.6e-05 -1.48128602308993e-09 0 0;-5.5e-05 -1.48162590680587e-09 0 0;-5.4e-05 -1.48196572160507e-09 0 0;-5.3e-05 -1.48230546742016e-09 0 0;-5.2e-05 -1.48264514418378e-09 0 0;-5.1e-05 -1.48298475182855e-09 0 0;-5e-05 -1.4833242902871e-09 0 0;-4.9e-05 -1.48366375949204e-09 -357.141627594736 -22168.6598365108;-4.8e-05 -1.48400315937599e-09 -349.004318568581 -22168.9603205432;-4.7e-05 -1.48434248987157e-09 -340.866844233413 -22169.2578060005;-4.6e-05 -1.48468175091137e-09 -332.729205697962 -22169.552292804;-4.5e-05 -1.485020942428e-09 -324.591404070993 -22169.8437808757;-4.4e-05 -1.48536006435407e-09 -316.453440461304 -22170.1322701376;-4.3e-05 -1.48569911662215e-09 -308.31531597773 -22170.4177605124;-4.2e-05 -1.48603809916485e-09 -300.177031729138 -22170.7002519231;-4.1e-05 -1.48637701191475e-09 -292.038588824429 -22170.979744293;-4e-05 -1.48671585480444e-09 -283.89998837254 -22171.2562375461;-3.9e-05 -1.48705462776648e-09 -275.761231482441 -22171.5297316065;-3.8e-05 -1.48739333073346e-09 -267.622319263134 -22171.8002263989;-3.7e-05 -1.48773196363795e-09 -259.483252823657 -22172.0677218484;-3.6e-05 -1.48807052641251e-09 -251.344033273082 -22172.3322178805;-3.5e-05 -1.48840901898971e-09 -243.204661720511 -22172.593714421;-3.4e-05 -1.4887474413021e-09 -235.06513927508 -22172.8522113962;-3.3e-05 -1.48908579328223e-09 -226.92546704596 -22173.1077087329;-3.2e-05 -1.48942407486267e-09 -218.785646142353 -22173.3602063581;-3.1e-05 -1.48976228597595e-09 -210.645677673494 -22173.6097041994;-3e-05 -1.49010042655462e-09 -202.505562748651 -22173.8562021847;-2.9e-05 -1.49043849653122e-09 -194.365302477123 -22174.0997002425;-2.8e-05 -1.49077649583827e-09 -186.224897968242 -22174.3401983013;-2.7e-05 -1.49111442440832e-09 -178.084350331372 -22174.5776962906;-2.6e-05 -1.49145228217389e-09 -169.94366067591 -22174.8121941397;-2.5e-05 -1.4917900690675e-09 -161.802830111283 -22175.0436917788;-2.4e-05 -1.49212778502168e-09 -153.661859746949 -22175.2721891381;-2.3e-05 -1.49246542996893e-09 -145.5207506924 -22175.4976861487;-2.2e-05 -1.49280300384177e-09 -137.379504057157 -22175.7201827416;-2.1e-05 -1.49314050657271e-09 -129.238120950773 -22175.9396788486;-2e-05 -1.49347793809425e-09 -121.096602482831 -22176.1561744017;-1.9e-05 -1.49381529833889e-09 -112.954949762947 -22176.3696693333;-1.8e-05 -1.49415258723913e-09 -104.813163900765 -22176.5801635763;-1.7e-05 -1.49448980472747e-09 -96.6712460059612 -22176.7876570641;-1.6e-05 -1.49482695073638e-09 -88.5291971882416 -22176.9921497304;-1.5e-05 -1.49516402519836e-09 -80.3870185573423 -22177.1936415092;-1.4e-05 -1.49550102804588e-09 -72.2447112230298 -22177.392132335;-1.3e-05 -1.49583795921143e-09 -64.1022762950993 -22177.5876221429;-1.2e-05 -1.49617481862747e-09 -55.9597148833777 -22177.7801108682;-1.1e-05 -1.49651160622649e-09 -47.8170280977188 -22177.9695984466;-1e-05 -1.49684832194094e-09 -39.6742170480088 -22178.1560848143;-9e-06 -1.49718496570329e-09 -31.531282844162 -22178.3395699078;-8e-06 -1.49752153744599e-09 -23.3882265961192 -22178.5200536643;-7e-06 -1.49785803710152e-09 -15.2450494138548 -22178.6975360211;-6e-06 -1.4981944646023e-09 -7.10175240736817 -22178.8720169159;-5e-06 -1.4985308198808e-09 1.04166331331044 -22179.0434962871;-4e-06 -1.49886710286946e-09 9.18519663812367 -22179.2119740733;-3e-06 -1.49920331350072e-09 17.3288464569846 -22179.3774502136;-2e-06 -1.49953945170701e-09 25.4726116597785 -22179.5399246473;-1e-06 -1.49987551742078e-09 33.6164911363639 -22179.6993973145]  x3=[-5.8e-05 -1.75936912022998e-11 0 0;-5.7e-05 -1.76159662568073e-11 0 0;-5.6e-05 -1.76382440213495e-11 0 0;-5.5e-05 -1.76605244943458e-11 0 0;-5.4e-05 -1.7682807674215e-11 0 0;-5.3e-05 -1.77050935593747e-11 0 0;-5.2e-05 -1.77273821482415e-11 0 0;-5.1e-05 -1.77496734392315e-11 0 0;-5e-05 -1.77719674307596e-11 0 0;-4.9e-05 -1.77942641212399e-11 -795.042090385786 1252.25715996356;-4.8e-05 -1.78165635090856e-11 -795.415586609114 1251.857000825;-4.7e-05 -1.78388655927089e-11 -795.788900429591 1251.4567318714;-4.6e-05 -1.78611703705213e-11 -796.162031815558 1251.05635318145;-4.5e-05 -1.78834778409332e-11 -796.53498073539 1250.65586483383;-4.4e-05 -1.79057880023542e-11 -796.907747157493 1250.25526690722;-4.3e-05 -1.79281008531931e-11 -797.280331050311 1249.85455948034;-4.2e-05 -1.79504163918575e-11 -797.652732382314 1249.45374263188;-4.1e-05 -1.79727346167545e-11 -798.024951122008 1249.05281644056;-4e-05 -1.79950555262899e-11 -798.396987237934 1248.65178098511;-3.9e-05 -1.80173791188689e-11 -798.768840698661 1248.25063634426;-3.8e-05 -1.80397053928957e-11 -799.140511472795 1247.84938259676;-3.7e-05 -1.80620343467736e-11 -799.511999528972 1247.44801982136;-3.6e-05 -1.8084365978905e-11 -799.883304835862 1247.04654809682;-3.5e-05 -1.81067002876913e-11 -800.254427362167 1246.64496750191;-3.4e-05 -1.81290372715333e-11 -800.625367076625 1246.24327811541;-3.3e-05 -1.81513769288305e-11 -800.996123948001 1245.8414800161;-3.2e-05 -1.81737192579818e-11 -801.366697945097 1245.43957328278;-3.1e-05 -1.81960642573851e-11 -801.737089036747 1245.03755799426;-3e-05 -1.82184119254375e-11 -802.107297191819 1244.63543422934;-2.9e-05 -1.82407622605349e-11 -802.47732237921 1244.23320206686;-2.8e-05 -1.82631152610727e-11 -802.847164567855 1243.83086158564;-2.7e-05 -1.82854709254451e-11 -803.216823726716 1243.42841286451;-2.6e-05 -1.83078292520457e-11 -803.586299824793 1243.02585598233;-2.5e-05 -1.83301902392668e-11 -803.955592831117 1242.62319101796;-2.4e-05 -1.83525538855002e-11 -804.324702714748 1242.22041805026;-2.3e-05 -1.83749201891365e-11 -804.693629444787 1241.81753715809;-2.2e-05 -1.83972891485656e-11 -805.062372990361 1241.41454842035;-2.1e-05 -1.84196607621764e-11 -805.430933320632 1241.01145191593;-2e-05 -1.84420350283569e-11 -805.799310404795 1240.60824772372;-1.9e-05 -1.84644119454943e-11 -806.167504212077 1240.20493592263;-1.8e-05 -1.84867915119749e-11 -806.535514711739 1239.80151659158;-1.7e-05 -1.85091737261839e-11 -806.903341873074 1239.39798980949;-1.6e-05 -1.85315585865058e-11 -807.27098566541 1238.9943556553;-1.5e-05 -1.85539460913242e-11 -807.638446058103 1238.59061420794;-1.4e-05 -1.85763362390218e-11 -808.005723020547 1238.18676554637;-1.3e-05 -1.85987290279801e-11 -808.372816522166 1237.78280974955;-1.2e-05 -1.86211244565803e-11 -808.739726532417 1237.37874689644;-1.1e-05 -1.86435225232021e-11 -809.106453020791 1236.97457706602;-1e-05 -1.86659232262247e-11 -809.472995956811 1236.57030033727;-9e-06 -1.86883265640262e-11 -809.839355310034 1236.16591678918;-8e-06 -1.8710732534984e-11 -810.205531050048 1235.76142650076;-7e-06 -1.87331411374743e-11 -810.571523146474 1235.35682955101;-6e-06 -1.87555523698727e-11 -810.937331568969 1234.95212601895;-5e-06 -1.87779662305537e-11 -811.302956287218 1234.54731598361;-4e-06 -1.88003827178911e-11 -811.668397270943 1234.14239952402;-3e-06 -1.88228018302576e-11 -812.033654489897 1233.73737671922;-2e-06 -1.88452235660252e-11 -812.398727913866 1233.33224764827;-1e-06 -1.88676479235648e-11 -812.763617512668 1232.92701239022]  x4=[-5.8e-05 1.57235207818061e-11 0 0;-5.7e-05 1.5745323162868e-11 0 0;-5.6e-05 1.57671283015519e-11 0 0;-5.5e-05 1.57889361963758e-11 0 0;-5.4e-05 1.58107468458566e-11 0 0;-5.3e-05 1.58325602485104e-11 0 0;-5.2e-05 1.58543764028524e-11 0 0;-5.1e-05 1.58761953073972e-11 0 0;-5e-05 1.5898016960658e-11 0 0;-4.9e-05 1.59198413611475e-11 814.879518930805 -1384.79835409657;-4.8e-05 1.59416685073774e-11 815.299491013028 -1384.39278766167;-4.7e-05 1.59634983978585e-11 815.719279304424 -1383.98709498734;-4.6e-05 1.59853310311008e-11 816.138883767487 -1383.58127615254;-4.5e-05 1.60071664056132e-11 816.558304364745 -1383.1753312363;-4.4e-05 1.6029004519904e-11 816.977541058758 -1382.76926031762;-4.3e-05 1.60508453724805e-11 817.396593812118 -1382.36306347552;-4.2e-05 1.6072688961849e-11 817.815462587453 -1381.95674078905;-4.1e-05 1.6094535286515e-11 818.23414734742 -1381.55029233724;-4e-05 1.61163843449832e-11 818.652648054712 -1381.14371819917;-3.9e-05 1.61382361357573e-11 819.070964672052 -1380.73701845388;-3.8e-05 1.61600906573403e-11 819.489097162198 -1380.33019318047;-3.7e-05 1.61819479082339e-11 819.90704548794 -1379.92324245803;-3.6e-05 1.62038078869394e-11 820.324809612101 -1379.51616636564;-3.5e-05 1.62256705919569e-11 820.742389497538 -1379.10896498244;-3.4e-05 1.62475360217858e-11 821.159785107137 -1378.70163838753;-3.3e-05 1.62694041749245e-11 821.576996403822 -1378.29418666006;-3.2e-05 1.62912750498706e-11 821.994023350547 -1377.88660987916;-3.1e-05 1.63131486451207e-11 822.410865910299 -1377.47890812399;-3e-05 1.63350249591707e-11 822.827524046098 -1377.07108147372;-2.9e-05 1.63569039905154e-11 823.243997720998 -1376.66313000752;-2.8e-05 1.63787857376488e-11 823.660286898083 -1376.25505380458;-2.7e-05 1.64006701990641e-11 824.076391540475 -1375.8468529441;-2.6e-05 1.64225573732536e-11 824.492311611321 -1375.43852750529;-2.5e-05 1.64444472587086e-11 824.908047073811 -1375.03007756736;-2.4e-05 1.64663398539196e-11 825.323597891159 -1374.62150320955;-2.3e-05 1.64882351573762e-11 825.738964026616 -1374.21280451109;-2.2e-05 1.65101331675672e-11 826.154145443466 -1373.80398155124;-2.1e-05 1.65320338829803e-11 826.569142105025 -1373.39503440927;-2e-05 1.65539373021026e-11 826.983953974642 -1372.98596316443;-1.9e-05 1.657584342342e-11 827.398581015698 -1372.57676789602;-1.8e-05 1.65977522454179e-11 827.813023191609 -1372.16744868333;-1.7e-05 1.66196637665804e-11 828.227280465824 -1371.75800560566;-1.6e-05 1.66415779853911e-11 828.641352801821 -1371.34843874234;-1.5e-05 1.66634949003324e-11 829.055240163116 -1370.93874817267;-1.4e-05 1.6685414509886e-11 829.468942513254 -1370.52893397601;-1.3e-05 1.67073368125328e-11 829.882459815816 -1370.11899623169;-1.2e-05 1.67292618067525e-11 830.295792034413 -1369.70893501908;-1.1e-05 1.67511894910242e-11 830.708939132692 -1369.29875041754;-1e-05 1.67731198638261e-11 831.121901074329 -1368.88844250646;-9e-06 1.67950529236353e-11 831.534677823037 -1368.47801136521;-8e-06 1.68169886689283e-11 831.94726934256 -1368.06745707319;-7e-06 1.68389270981805e-11 832.359675596674 -1367.65677970983;-6e-06 1.68608682098665e-11 832.771896549192 -1367.24597935454;-5e-06 1.688281200246e-11 833.183932163953 -1366.83505608674;-4e-06 1.69047584744339e-11 833.595782404835 -1366.42400998588;-3e-06 1.69267076242601e-11 834.007447235747 -1366.01284113142;-2e-06 1.69486594504098e-11 834.418926620632 -1365.6015496028;-1e-06 1.6970613951353e-11 834.830220523462 -1365.19013547951]  x5=5.70973484498186e-05  V1=ones(3,3)  V2=ones(3,3)  I1=ones(3,3)  I2=ones(3,3)  nHarmo=1  Measurements=None
      settings: SourceProductName=Simscape Electrical
  2-MW Load : powerlib/Elements/Three-Phase Parallel RLC Load  LConnTagsString=A|B|C  Configuration=Y (grounded)  NominalVoltage=25e3  Vabc=[1e3 1e3 1e3]  Vabcp=[1e3 1e3 1e3]  NominalFrequency=60  UnbalancedPower=off  ActivePower=2e6  InductivePower=0  CapacitivePower=0  Pabc=[10e3 9e3 11e3]  QLabc=[100 90 110]  QCabc=[100 90 110]  Pabcp=[10e3 9e3 11e3]  QLabcp=[100 90 110]  QCabcp=[100 90 110]  Measurements=None  LoadType=constant Z
      settings: SourceProductName=Simscape Electrical
  "3.3ohms " : powerlib/Elements/Series RLC Branch  LConnTagsString=__new0  RConnTagsString=__new0  BranchType=R  Resistance=3.3  Inductance=[]  SetiL0=off  InitialCurrent=0  Capacitance=[]  Setx0=off  InitialVoltage=0  Measurements=None
      settings: SourceProductName=Simscape Electrical
  30-MW 2-Mvar Load : powerlib/Elements/Three-Phase Parallel RLC Load  LConnTagsString=A|B|C  Configuration=Y (grounded)  NominalVoltage=25e3  Vabc=[1e3 1e3 1e3]  Vabcp=[1e3 1e3 1e3]  NominalFrequency=60  UnbalancedPower=off  ActivePower=30e6  InductivePower=2e6  CapacitivePower=0  Pabc=[10e3 9e3 11e3]  QLabc=[100 90 110]  QCabc=[100 90 110]  Pabcp=[10e3 9e3 11e3]  QLabcp=[100 90 110]  QCabcp=[100 90 110]  Measurements=None  LoadType=constant Z
      settings: SourceProductName=Simscape Electrical
  5-km Feeder : powerlib/Elements/Distributed Parameters Line  Phases=3  Frequency=60  Resistance=[0.1153 0.413]  Inductance=[1.05e-3 3.32e-3]  Capacitance=[11.33e-009 5.01e-009]  Length=5  x1=[-2.1e-05 -2.40008256312818e-14 9569.17740195213 -16829.7487756047;-2e-05 -2.28579445886096e-14 9574.46415115671 -16826.7416993967;-1.9e-05 -2.17150612899488e-14 9579.74995539955 -16823.7329624558;-1.8e-05 -2.05721758480973e-14 9585.03481415899 -16820.7225650791;-1.7e-05 -1.94292883758534e-14 9590.31872691341 -16817.7105075636;-1.6e-05 -1.82863989860156e-14 9595.60169314132 -16814.6967902066;-1.5e-05 -1.71435077913827e-14 9600.88371232131 -16811.6814133056;-1.4e-05 -1.60006149047533e-14 9606.16478393207 -16808.6643771581;-1.3e-05 -1.48577204389266e-14 9611.44490745238 -16805.645682062;-1.2e-05 -1.37148245067016e-14 9616.7240823611 -16802.6253283151;-1.1e-05 -1.25719272208777e-14 9622.00230813721 -16799.6033162156;-1e-05 -1.14290286942544e-14 9627.27958425976 -16796.5796460617;-9e-06 -1.02861290396311e-14 9632.55591020791 -16793.5543181519;-8e-06 -9.14322836980764e-15 9637.8312854609 -16790.5273327847;-7e-06 -8.00032679758369e-15 9643.10570949808 -16787.4986902589;-6e-06 -6.85742443575914e-15 9648.37918179889 -16784.4683908734;-5e-06 -5.71452139713394e-15 9653.65170184285 -16781.4364349273;-4e-06 -4.57161779450808e-15 9658.92326910957 -16778.4028227199;-3e-06 -3.42871374068163e-15 9664.1938830788 -16775.3675545504;-2e-06 -2.2858093484547e-15 9669.46354323032 -16772.3306307185;-1e-06 -1.14290473062744e-15 9674.73224904406 -16769.292051524]  x2=[-2.1e-05 -3.41085825404493e-10 6932.68714853599 -18239.2100187145;-2e-05 -3.4117135551319e-10 6938.72534872768 -18237.0791150938;-1.9e-05 -3.41256874037133e-10 6944.76289723849 -18234.9461983069;-1.8e-05 -3.4134238095955e-10 6950.79979339215 -18232.8112685519;-1.7e-05 -3.41427876263664e-10 6956.83603651243 -18230.674326027;-1.6e-05 -3.41513359932698e-10 6962.87162592319 -18228.5353709308;-1.5e-05 -3.41598831949874e-10 6968.90656094833 -18226.3944034619;-1.4e-05 -3.41684292298408e-10 6974.94084091182 -18224.2514238192;-1.3e-05 -3.41769740961519e-10 6980.97446513768 -18222.1064322021;-1.2e-05 -3.41855177922421e-10 6987.00743295 -18219.9594288098;-1.1e-05 -3.41940603164327e-10 6993.03974367293 -18217.810413842;-1e-05 -3.42026016670447e-10 6999.07139663066 -18215.6593874985;-9e-06 -3.4211141842399e-10 7005.10239114747 -18213.5063499795;-8e-06 -3.42196808408162e-10 7011.13272654769 -18211.3513014853;-7e-06 -3.4228218660617e-10 7017.1624021557 -18209.1942422164;-6e-06 -3.42367553001215e-10 7023.19141729595 -18207.0351723736;-5e-06 -3.42452907576499e-10 7029.21977129294 -18204.8740921578;-4e-06 -3.42538250315221e-10 7035.24746347125 -18202.7110017705;-3e-06 -3.42623581200577e-10 7041.27449315551 -18200.5459014129;-2e-06 -3.42708900215763e-10 7047.3008596704 -18198.3787912868;-1e-06 -3.42794207343972e-10 7053.32656234069 -18196.2096715941]  x3=[-2.1e-05 -1.40495251629074e-11 -820.621321245342 1305.86571313749;-2e-05 -1.40684867761517e-11 -821.01203357342 1305.45778473352;-1.9e-05 -1.40874512242091e-11 -821.402561158518 1305.04974096463;-1.8e-05 -1.41064185060077e-11 -821.792903967184 1304.6415819102;-1.7e-05 -1.41253886204748e-11 -822.183061965993 1304.2333076496;-1.6e-05 -1.41443615665368e-11 -822.573035121558 1303.82491826223;-1.5e-05 -1.41633373431192e-11 -822.962823400522 1303.41641382749;-1.4e-05 -1.41823159491467e-11 -823.352426769564 1303.00779442477;-1.3e-05 -1.4201297383543e-11 -823.741845195392 1302.59906013351;-1.2e-05 -1.4220281645231e-11 -824.13107864475 1302.19021103312;-1.1e-05 -1.42392687331327e-11 -824.520127084415 1301.78124720303;-1e-05 -1.42582586461692e-11 -824.908990481193 1301.37216872271;-9e-06 -1.42772513832608e-11 -825.297668801928 1300.96297567159;-8e-06 -1.42962469433269e-11 -825.686162013496 1300.55366812915;-7e-06 -1.43152453252859e-11 -826.074470082804 1300.14424617486;-6e-06 -1.43342465280553e-11 -826.462592976793 1299.7347098882;-5e-06 -1.4353250550552e-11 -826.850530662436 1299.32505934866;-4e-06 -1.43722573916918e-11 -827.238283106742 1298.91529463574;-3e-06 -1.43912670503896e-11 -827.62585027675 1298.50541582896;-2e-06 -1.44102795255594e-11 -828.013232139533 1298.09542300783;-1e-06 -1.44292948161147e-11 -828.400428662198 1297.68531625188]  x4=[-2.1e-05 1.20870585182036e-11 874.430637002339 -1421.04510289624;-2e-05 1.21062018298888e-11 874.858542868276 -1420.62042473868;-1.9e-05 1.21253481612795e-11 875.286258787791 -1420.19561915099;-1.8e-05 1.21444975112934e-11 875.713784723495 -1419.77068621415;-1.7e-05 1.21636498788472e-11 876.141120638033 -1419.34562600917;-1.6e-05 1.21828052628567e-11 876.568266494083 -1418.92043861703;-1.5e-05 1.22019636622369e-11 876.995222254357 -1418.49512411877;-1.4e-05 1.22211250759019e-11 877.4219878816 -1418.06968259539;-1.3e-05 1.22402895027646e-11 877.848563338591 -1417.64411412795;-1.2e-05 1.22594569417375e-11 878.274948588141 -1417.21841879748;-1.1e-05 1.22786273917318e-11 878.701143593096 -1416.79259668505;-1e-05 1.22978008516579e-11 879.127148316335 -1416.36664787171;-9e-06 1.23169773204255e-11 879.552962720772 -1415.94057243856;-8e-06 1.23361567969431e-11 879.978586769352 -1415.51437046668;-7e-06 1.23553392801186e-11 880.404020425055 -1415.08804203716;-6e-06 1.23745247688587e-11 880.829263650894 -1414.66158723113;-5e-06 1.23937132620694e-11 881.254316409915 -1414.23500612969;-4e-06 1.24129047586559e-11 881.679178665198 -1413.80829881399;-3e-06 1.24320992575222e-11 882.103850379859 -1413.38146536517;-2e-06 1.24512967575716e-11 882.528331517042 -1412.95450586437;-1e-06 1.24704972577066e-11 882.95262203993 -1412.52742039277]  x5=2.03919101606495e-05  V1=ones(3,3)  V2=ones(3,3)  I1=ones(3,3)  I2=ones(3,3)  nHarmo=1  Measurements=None
      settings: SourceProductName=Simscape Electrical
  Ground3 : powerlib/Elements/Ground  LConnTagsString=a
      settings: SourceProductName=Simscape Electrical
  "Grounding Transformer " : powerlib/Elements/Grounding Transformer   UNITS=pu  NominalPower="[100e6   60]"  NominalVoltage=25e3  ZeroSequenceImpedance_pu=[0.025 0.75]  MagnetizationBranch_pu=[500 500]  ZeroSequenceImpedance_SI=[0.052083 589.05]  MagnetizationBranch_SI=[1041.7 3.927e+005]  Measurements=None
      settings: SourceProductName=Simscape Electrical  SourceProductBaseCode=PS
  A : PMIOPort  Side=Left
  B : PMIOPort  Port=2  Side=Left
  C : PMIOPort  Port=3  Side=Left
  connections:
  "3.3ohms "/RConn1 -- Ground3/LConn1
  120 kV / 25 kV 47 MVA/LConn1 -- 120kV 2500MVA/RConn1
  120 kV / 25 kV 47 MVA/LConn2 -- 120kV 2500MVA/RConn2
  120 kV / 25 kV 47 MVA/LConn3 -- 120kV 2500MVA/RConn3
  120 kV / 25 kV 47 MVA/RConn1 -- "Grounding Transformer "/LConn1 -- 14-km Feeder/RConn1 -- 30-MW 2-Mvar Load/LConn1
  120 kV / 25 kV 47 MVA/RConn2 -- "Grounding Transformer "/LConn2 -- 14-km Feeder/RConn2 -- 30-MW 2-Mvar Load/LConn2
  120 kV / 25 kV 47 MVA/RConn3 -- "Grounding Transformer "/LConn3 -- 14-km Feeder/RConn3 -- 30-MW 2-Mvar Load/LConn3
  5-km Feeder/RConn1 -- 14-km Feeder/LConn1 -- 2-MW Load/LConn1
  5-km Feeder/RConn2 -- 14-km Feeder/LConn2 -- 2-MW Load/LConn2
  5-km Feeder/RConn3 -- 14-km Feeder/LConn3 -- 2-MW Load/LConn3
  A/RConn1 -- 5-km Feeder/LConn1
  B/RConn1 -- 5-km Feeder/LConn2
  C/RConn1 -- 5-km Feeder/LConn3
  "Grounding Transformer "/RConn1 -- "3.3ohms "/LConn1

== system Hybrid_PV_Wind_Subsystem/Pmean1 ==
  Product : Product  RndMeth=Zero
  WkW : Gain  Gain=1/1000
  P : Outport
  V : Outport  Port=2
  wires:
  [Vmean_PV] -> Product/1, V/1
  Product/1 -> WkW/1
  [Imean_PV] -> Product/2
  WkW/1 -> P/1  "Pmean_PV (kW)"

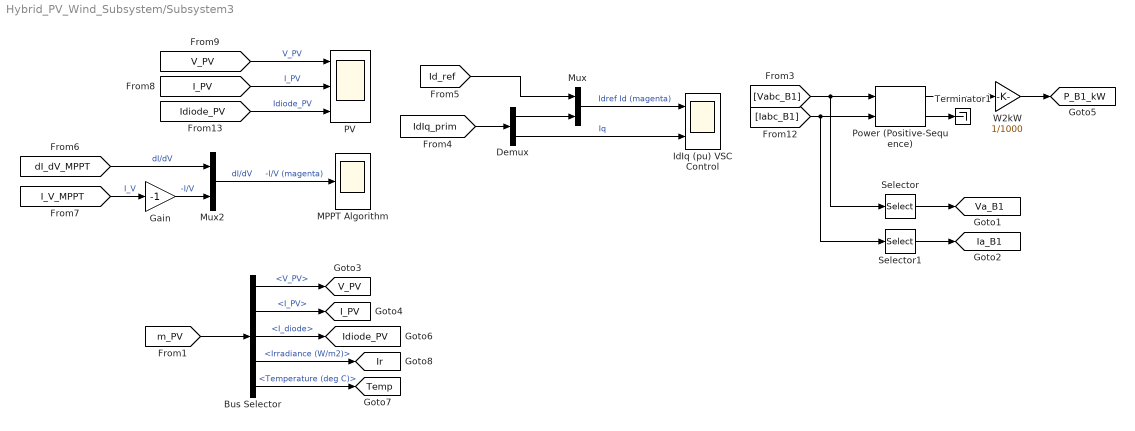
== system Hybrid_PV_Wind_Subsystem/Subsystem3 ==
  Bus Selector : BusSelector  OutputSignals=V_PV,I_PV,I_diode,Irradiance (W/m2),Temperature (deg C)
  Demux : Demux  Outputs=2
  Gain : Gain  Gain=-1
  IdIq (pu) VSC Control : Scope  NumInputPorts=2
  MPPT Algorithm : Scope
  Mux : Mux  Inputs=2
  Mux2 : Mux  Inputs=2
  PV : Scope  NumInputPorts=3
  Power (Positive-Sequence) : powerlib_meascontrol/Measurements/Power (Positive-Sequence)  Freq=60  Vinit=[0, 0]  Iinit=[0, 0]  Ts=Ts_Control
      settings: SourceProductName=Simscape Electrical  SourceProductBaseCode=PS
  Selector : Selector  InputPortWidth=3  IndexOptions=Index vector (dialog)  Indices=[1]  OutputSizes=1
  Selector1 : Selector  InputPortWidth=3  IndexOptions=Index vector (dialog)  Indices=[1]  OutputSizes=1
  Terminator1 : Terminator
  W2kW : Gain  Gain=1/1000
  tag scope: I_PV=global, Ia_B1=global, Idiode_PV=global, Ir=global, P_B1_kW=global, Temp=global, V_PV=global, Va_B1=global
  wires:
  [Vabc_B1] -> Power (Positive-Sequence)/1, Selector/1
  [Iabc_B1] -> Power (Positive-Sequence)/2, Selector1/1
  Power (Positive-Sequence)/1 -> W2kW/1
  [I_V_MPPT] -> Gain/1  "I_V"
  [IdIq_prim] -> Demux/1
  [Id_ref] -> Mux/1
  Demux/1 -> Mux/2
  Mux/1 -> IdIq (pu) VSC Control/1  "Idref Id (magenta)"
  Demux/2 -> IdIq (pu) VSC Control/2  "Iq"
  Selector/1 -> [Va_B1]
  Selector1/1 -> [Ia_B1]
  [V_PV] -> PV/1  "V_PV"
  [I_PV] -> PV/2  "I_PV"
  [Idiode_PV] -> PV/3  "Idiode_PV"
  [dI_dV_MPPT] -> Mux2/1  "dI/dV"
  Gain/1 -> Mux2/2  "-I/V"
  Mux2/1 -> MPPT Algorithm/1  "dI/dV     -I/V (magenta)"
  W2kW/1 -> [P_B1_kW]
  [m_PV] -> Bus Selector/1
  Bus Selector/1 -> [V_PV]  "<V_PV>"
  Bus Selector/2 -> [I_PV]  "<I_PV>"
  Bus Selector/4 -> [Ir]  "<Irradiance (W/m2)>"
  Bus Selector/3 -> [Idiode_PV]  "<I_diode>"
  Bus Selector/5 -> [Temp]  "<Temperature (deg C)>"
  Power (Positive-Sequence)/2 -> Terminator1/1

== system Hybrid_PV_Wind_Subsystem/Subsystem4 ==
  Mean : powerlib_meascontrol/Measurements/Mean  Freq=60  Vinit=0  Ts=Ts_Control
      settings: SourceProductName=Simscape Electrical
  Mux1 : Mux  Inputs=2
  Vm : Outport
  VrVm : Outport  Port=2
  wires:
  [Vdc_ref] -> Mux1/1  "Vdc ref"
  [Vdc] -> Mean/1  "Vdc"
  Mux1/1 -> VrVm/1
  Mean/1 -> Mux1/2, Vm/1

== system Hybrid_PV_Wind_Subsystem/ Modul PV Array Power System/Irradiance Temp ==
  Demux : Demux  Tag=STV Demux  Outputs=2
  FromWs : FromWorkspace  Tag=STV FromWs  VariableName=tuvar  SampleTime=0
      SigBuilderData=|
      | common.afterFinalStr = 'Extrapolate'
      | common.sampleTime = '0'
      | dataSet(1).timeRange = [0 2]
      | dataSet(1).name = 'Constant Irradiance'
      | dataSet(2).timeRange = [0 2]
      | dataSet(2).name = 'Step Irradiance'
      | dataSet(3).timeRange = [0 10]
      | dataSet(3).name = 'Ramp-up/down Irradiance'
      | sbobj.Groups(1).Name = 'Constant Irradiance'
      | sbobj.Groups(1).Signals(1).Name = 'Ir'
      | sbobj.Groups(1).Signals(1).XData = [0 2]
      | sbobj.Groups(1).Signals(1).YData = [1000 1000]
      | sbobj.Groups(1).Signals(2).Name = 'Temp'
      | sbobj.Groups(1).Signals(2).XData = [0 1 1 2]
      | sbobj.Groups(1).Signals(2).YData = [0 0 1 1]
      | sbobj.Groups(1).TimeRange = [0 2]
      | sbobj.Groups(2).Name = 'Step Irradiance'
      | sbobj.Groups(2).Signals(1).Name = 'Ir'
      | sbobj.Groups(2).Signals(1).XData = [0 0.252 0.252 2]
      | sbobj.Groups(2).Signals(1).YData = [600 600 1000 1000]
      | sbobj.Groups(2).Signals(2).Name = 'Temp'
      | sbobj.Groups(2).Signals(2).XData = [0 1 1 2]
      | sbobj.Groups(2).Signals(2).YData = [0 0 1 1]
      | sbobj.Groups(2).TimeRange = [0 2]
      | sbobj.Groups(3).Name = 'Ramp-up/down Irradiance'
      | sbobj.Groups(3).Signals(1).Name = 'Ir'
      | sbobj.Groups(3).Signals(1).XData = [0 3 4.7 5 6.6 10]
      | sbobj.Groups(3).Signals(1).YData = [1000 1000 250 250 1000 1000]
      | sbobj.Groups(3).Signals(2).Name = 'Temp'
      | sbobj.Groups(3).Signals(2).XData = [0 6 6.4 10]
      | sbobj.Groups(3).Signals(2).YData = [25 25 50 50]
  Ir : Outport  Tag=STV Outport
  Temp : Outport  Tag=STV Outport  Port=2
  wires:
  Demux/1 -> Ir/1
  FromWs/1 -> Demux/1
  Demux/2 -> Temp/1

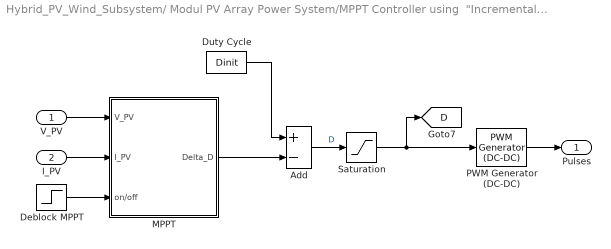
== system Hybrid_PV_Wind_Subsystem/ Modul PV Array Power System/MPPT Controller using  "Incremental Conductance + Integral Regulator "  technique  ==
  V_PV : Inport
  I_PV : Inport  Port=2
  Add : Sum  Inputs=+-
  Deblock MPPT : Step  Time=0.4  SampleTime=0
  Duty Cycle : Constant  Value=Dinit
  MPPT : Subsystem
  PWM Generator (DC-DC) : powerlib_meascontrol/Pulse & Signal Generators/PWM Generator (DC-DC)  Fsw=fc  Ts=Ts_Power
      settings: SourceProductName=Simscape Electrical
  Saturation : Saturate  UpperLimit=1  LowerLimit=0
  Pulses : Outport
  tag scope: D=global
  wires:
  V_PV/1 -> MPPT/1(V_PV)
  I_PV/1 -> MPPT/2(I_PV)
  PWM Generator (DC-DC)/1 -> Pulses/1
  Deblock MPPT/1 -> MPPT/3(on/off)
  Saturation/1 -> PWM Generator (DC-DC)/1, [D]
  Add/1 -> Saturation/1  "D"
  MPPT/1(Delta_D) -> Add/2
  Duty Cycle/1 -> Add/1
